simulink model "SWING_UP_ENERGY_BASED_plus_PP"  (R2022b)
settings: Solver=FixedStepAuto  StartTime=0.0  StopTime=inf  FixedStep=0.002  RelTol=1e-3  EnableMultiTasking=on
undefined symbols (not defined in the file or in its folder): A, B, C, D, g0, HIL, Ip, K, K_pp, L_kf, Lp, Lr, mp, mr, qc_get_step_size, Ra
libraries: quarc_library x8, simulink_extras x7
settings Model: ExtModeTrigDuration=10000  Creator=Utente  LastModifiedBy=Utente
settings SolverCC: AlgebraicLoopSolver=TrustRegion  PositivePriorityOrder=on
settings DataIOCC: ReturnWorkspaceOutputs=off
settings DebuggingCC: UnconnectedInputMsg=warning  UnconnectedOutputMsg=warning  UnconnectedLineMsg=warning  SFMachineParentedDataDiag=warning  ArithmeticOperatorsInVariantConditions=warning
settings ModelReferenceCC: EnableRefExpFcnMdlSchedulingChecks=on
settings SFSimCC: SimUseLocalCustomCode=off  CustomCodeUndefinedFunction=UseInterfaceOnly
settings RTWCC: Description=QUARC Win64 Target Using Toolchain  SystemTargetFile=quarc_win64.tlc  TemplateMakefile=quarc_default_tmf  RTWUseLocalCustomCode=off  Toolchain=QUARC win64 | nmake (64-bit Windows)  BuildConfiguration=Faster Runs
settings CodeAppCC: StateflowObjectComments=on
settings STFCustomTargetCC: TargetLangStandard=C99 (ISO)  ConcurrentExecutionCompliant=on  GRTInterface=on  UseToolchainInfoCompliant=on  SystemTargetFile=quarc_win64.tlc
settings GRTTargetCC: ParMdlRefBuildCompliant=off  CompOptLevelCompliant=off  CombineOutputUpdateFcns=off  MatFileLogging=off  CPPClassGenCompliant=off  GRTInterface=on  ExtMode=on  ExtModeMexFile=quarc_comm
settings ConfigComp: CovMetricSettings=dswe

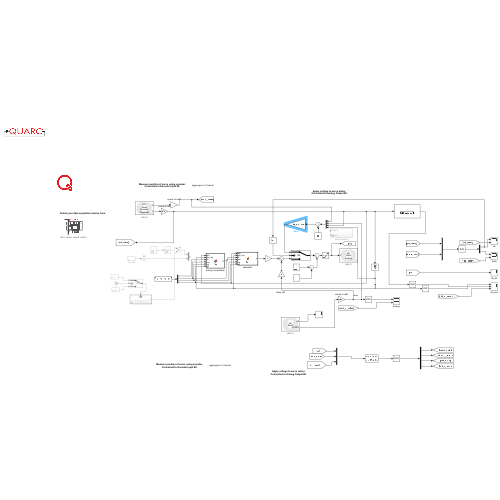
[thumbnail: Simulink's stored preview of the top-level diagram]
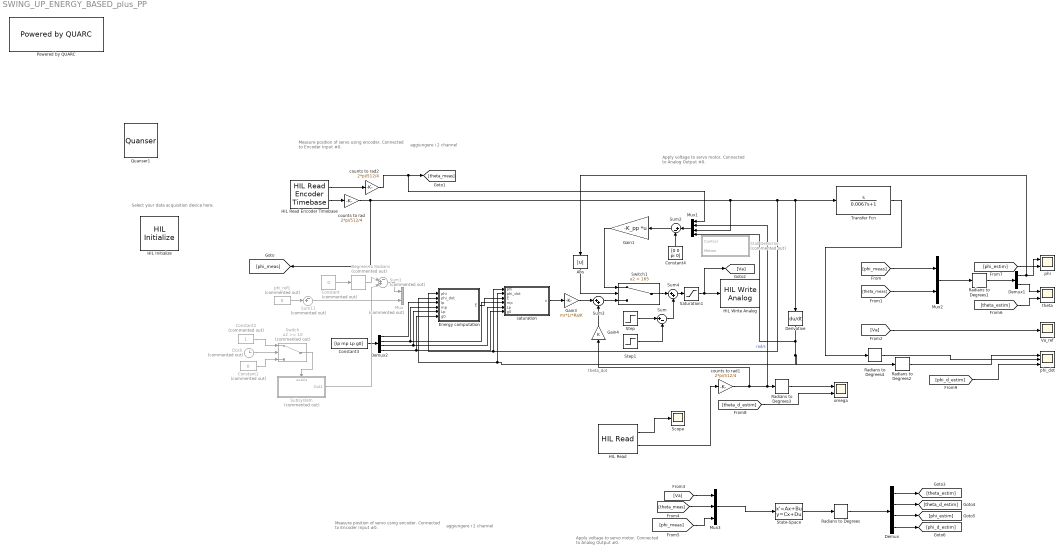
== system SWING_UP_ENERGY_BASED_plus_PP ==
  note: theta_dot
  note: aggiungere i 2 channel
  note: Apply voltage to servo motor.
      | Connected to Analog Output #0.
  note: Measure position of servo using encoder.
      | Connected to Encoder Input #0.
  note: aggiungere i 2 channel
  note: Measure position of servo using encoder.
      | Connected to Encoder Input #0.
  note: Apply voltage to servo motor.
      | Connected to Analog Output #0.
  note: Select your data acquisition device here.
  Abs : Abs  SaturateOnIntegerOverflow=off
  Clock : Clock  Commented=on
  Constant : Constant  Commented=on  Value=0
  Constant1 : Constant  Commented=on  Value=0
  Constant2 : Constant  Commented=on
  Constant3 : Constant  Value=[Ip mp Lp g0]
  Constant4 : Constant  Value=[0 0 pi 0]
  Degrees to Radians : simulink_extras/Transformations/Degrees to Radians  Commented=on
  Demux : Demux
  Demux1 : Demux  Outputs=2
  Demux2 : Demux
  Derivative : Derivative
  Energy computation : MATLAB Function  TreatAsAtomicUnit=on
  Gain1 : Gain  Gain=-K_pp  Multiplication=Matrix(K*u) (u vector)
  Gain3 : Gain  Gain=mr*Lr*Ra/K
  Gain4 : Gain  Gain=K
  HIL Initialize : quarc_library/Data Acquisition/Generic/Configuration/HIL Initialize  Priority=-99  object_name=HIL-1  board_type=qube_servo2_usb  board_number=0  board_options=""  exclusive=off  active=off  hardware_clocks=[0]  clock_modes=[]  initial_clock_frequencies=[]  set_clock_params_at_start=off  set_clock_params_at_switch_in=off  set_clock_frequencies_at_start=off  set_clock_frequencies_at_switch_in=off  analog_input_channels=[0]  analog_input_configurations=[]  analog_input_maximums=3  analog_input_minimums=-3  set_analog_input_params_at_start=off  set_analog_input_params_at_switch_in=off  analog_output_channels=[0]  analog_output_maximums=15  analog_output_minimums=-15  initial_analog_outputs=[0]  final_analog_outputs=[0]  watchdog_analog_outputs=0  set_analog_output_params_at_start=off  set_analog_output_params_at_switch_in=off  set_analog_outputs_at_start=on  set_analog_outputs_at_switch_in=off  set_analog_outputs_at_terminate=on  set_analog_outputs_at_switch_out=off  set_analog_outputs_on_watchdog=on  digital_input_channels=[]  digital_output_channels=[0]  digital_output_configuration=[]  initial_digital_outputs=[1]  final_digital_outputs=[0]  watchdog_digital_outputs=[0]  set_digital_output_params_at_start=off  set_digital_output_params_at_switch_in=off  set_digital_outputs_at_start=on  set_digital_outputs_at_switch_in=off  set_digital_outputs_at_terminate=on  set_digital_outputs_at_switch_out=off  set_digital_outputs_on_watchdog=on  encoder_channels=[0:1]  quadrature=[4]  encoder_filter_frequency=[]  initial_encoder_counts=[0]  set_encoder_params_at_start=off  set_encoder_params_at_switch_in=off  set_encoder_counts_at_start=on  set_encoder_counts_at_switch_in=off  pwm_channels=[]  pwm_modes=[]  pwm_frequency=[]  pwm_configuration=[]  pwm_alignment=[]  pwm_polarity=[]  pwm_leading_deadband=[]  pwm_trailing_deadband=[]  initial_pwm_outputs=[]  final_pwm_outputs=[]  watchdog_pwm_outputs=[]  set_pwm_params_at_start=off  set_pwm_params_at_switch_in=off  set_pwm_outputs_at_start=off  set_pwm_outputs_at_switch_in=off  set_pwm_outputs_at_terminate=off  set_pwm_outputs_at_switch_out=off  set_pwm_outputs_on_watchdog=off  other_output_channels=[11000:11002]  initial_other_outputs=[0 1 0]  final_other_outputs=[1 0 0]  watchdog_other_outputs=[0 0 1]  set_other_outputs_at_start=on  set_other_outputs_at_switch_in=off  set_other_outputs_at_terminate=on  set_other_outputs_at_switch_out=off  set_other_outputs_on_watchdog=on
  HIL Read : quarc_library/Data Acquisition/Generic/Immediate I//O/HIL Read  object_name=HIL-1  analog_channels=[0]  encoder_channels=[]  digital_channels=[]  other_channels=[14000]  sample_time=qc_get_step_size  active=on  vector_output=off  data_type_mode=Inherit via back propagation  encoder_data_type=double  digital_data_type=boolean
  HIL Read Encoder Timebase : quarc_library/Data Acquisition/Generic/Timebases/HIL Read Encoder Timebase  object_name=HIL-1  clock=0  channels=[0:1]  active=on  vector_output=off  data_type_mode=Inherit via back propagation  data_type=double  overflow_mode=Error on overflow  samples_in_buffer=max(ceil(1/qc_get_step_size), 1)
  HIL Write Analog : quarc_library/Data Acquisition/Generic/Immediate I//O/HIL Write Analog  object_name=HIL-1  channels=[0]  sample_time=-1  active=off  vector_input=off
  Mux : Mux  Commented=on  Inputs=2
  Mux1 : Mux
  Mux2 : Mux  Inputs=2
  Mux3 : Mux  Inputs=3
  Powered by QUARC : quarc_library/Logos/Powered by QUARC
  Quanser1 : quarc_library/Logos/Quanser
  Radians to Degrees{,1..4} (5 alike) : simulink_extras/Transformations/Radians to Degrees
  Saturation1 : Saturate  UpperLimit=10  LowerLimit=-10
  Scope : Scope
  Stall Detection : Subsystem  Commented=on
  State-Space : StateSpace  A=A-L_kf*C  B=[B-L_kf*D L_kf]  C=eye(4)  D=zeros(4,3)  InitialCondition=0
  Step : Step  SampleTime=0
  Step1 : Step  Time=1.001  SampleTime=0
  Subsystem : Subsystem  Commented=on
  Sum : Sum  Inputs=|+-
  Sum1 : Sum  Commented=on  Inputs=-++|
  Sum11 : Sum  Commented=on  Inputs=-+|
  Sum2 : Sum  Inputs=|+-
  Sum3 : Sum  Inputs=|++
  Sum4 : Sum  Inputs=|++
  Switch : Switch  Commented=on  Threshold=10  SaturateOnIntegerOverflow=off  InputSameDT=off
  Switch1 : Switch  Criteria=u2 > Threshold  Threshold=165  SaturateOnIntegerOverflow=off  InputSameDT=off
  Transfer Fcn : TransferFcn  Numerator=[1 0]  Denominator=[0.0067 1]
  Va_ref : Scope
  counts to rad : Gain  Gain=2*pi/512/4
  counts to rad1 : Gain  Gain=2*pi/512/4
  counts to rad2 : Gain  Gain=2*pi/512/4
  omega : Scope  NumInputPorts=2
  phi : Scope  NumInputPorts=2
  phi_dot : Scope  NumInputPorts=3
  phi_ref1 : Constant  Commented=on  Value=0
  saturation : MATLAB Function  TreatAsAtomicUnit=on
  theta : Scope  NumInputPorts=2
  wires:
  [Va] -> Mux3/1
  Demux2/3 -> saturation/5(Lp), Energy computation/5(Lp)
  Demux2/2 -> saturation/4(mp), Energy computation/4(mp)
  saturation/1(u) -> Gain3/1
  Radians to Degrees3/1 -> omega/1
  Demux2/4 -> Energy computation/6(g0), saturation/6(g0)
  Demux2/1 -> Energy computation/3(Ip)
  counts to rad2/1 -> Mux1/1, [theta_meas]
  Radians to Degrees1/1 -> Demux1/1
  Constant3/1 -> Demux2/1
  counts to rad/1 -> [phi_meas], Mux1/3, Energy computation/1(phi), saturation/1(phi), Derivative/1, Transfer Fcn/1
  Energy computation/1(E) -> saturation/3(E)
  Clock/1 -> Switch/2
  Demux/1 -> [theta_estim]
  Gain4/1 -> Sum3/2
  Saturation1/1 -> [Va], HIL Write Analog/1
  Constant1/1 -> Switch/3
  Switch/1 -> Subsystem/Enable
  Sum1/1 -> Mux/1
  Radians to Degrees4/1 -> phi_dot/2
  Demux/3 -> [phi_estim]
  [phi_d_estim] -> phi_dot/3
  [phi_meas] -> Mux3/3
  [theta_d_estim] -> omega/2
  [theta_estim] -> theta/2
  HIL Read/2 -> counts to rad1/1
  Radians to Degrees2/1 -> phi_dot/1
  [theta_meas] -> Mux3/2
  Demux1/2 -> theta/1
  HIL Read/1 -> Scope/1
  Constant/1 -> Degrees to Radians/1
  [theta_meas] -> Mux2/2
  Transfer Fcn/1 -> Radians to Degrees4/1
  Degrees to Radians/1 -> Sum1/2
  Demux1/1 -> Abs/1, phi/1
  State-Space/1 -> Radians to Degrees/1
  Sum11/1 -> Mux/2
  [phi_meas] -> Mux2/1
  Mux2/1 -> Radians to Degrees1/1
  phi_ref1/1 -> Sum11/2
  Subsystem/1(Out1) -> Sum1/3
  Constant2/1 -> Switch/1
  Mux3/1 -> State-Space/1
  HIL Read Encoder Timebase/1 -> counts to rad2/1
  Demux/4 -> [phi_d_estim]
  [phi_estim] -> phi/2
  [Va] -> Va_ref/1
  Radians to Degrees/1 -> Demux/1
  Derivative/1 -> Mux1/4, Energy computation/2(phi_dot), saturation/2(phi_dot), Radians to Degrees2/1
  counts to rad1/1 -> Gain4/1, Mux1/2, Radians to Degrees3/1  "rad/s"
  Demux/2 -> [theta_d_estim]
  Gain3/1 -> Sum3/1
  HIL Read Encoder Timebase/2 -> counts to rad/1
  Abs/1 -> Switch1/2
  Sum3/1 -> Switch1/3
  Sum2/1 -> Gain1/1
  Constant4/1 -> Sum2/2
  Gain1/1 -> Switch1/1
  Mux1/1 -> Sum2/1
  Step/1 -> Sum/1
  Step1/1 -> Sum/2
  Sum4/1 -> Saturation1/1
  Switch1/1 -> Sum4/1
  Sum/1 -> Sum4/2

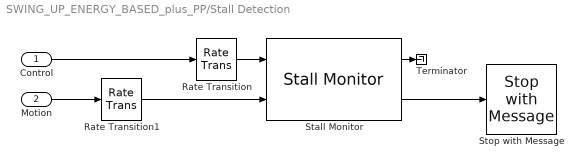
== system SWING_UP_ENERGY_BASED_plus_PP/Stall Detection ==
  Control : Inport
  Motion : Inport  Port=2
  Rate Transition : RateTransition
  Rate Transition1 : RateTransition
  Stall Monitor : quarc_library/Discrete/Stall Monitor  control_threshold=5  motion_threshold=0.3  duration_s=20
      settings: SourceProductName=QUARC Targets
  Stop with Message : quarc_library/Sinks/Error Handling/Stop with Message  message_type=Fixed error message  message_icon=Error  message=Stall Detected! Please ensure that the DC motor is free to move and is functioning properly
  Terminator : Terminator
  wires:
  Control/1 -> Rate Transition/1
  Motion/1 -> Rate Transition1/1
  Stall Monitor/2 -> Stop with Message/1
  Stall Monitor/1 -> Terminator/1
  Rate Transition/1 -> Stall Monitor/1
  Rate Transition1/1 -> Stall Monitor/2

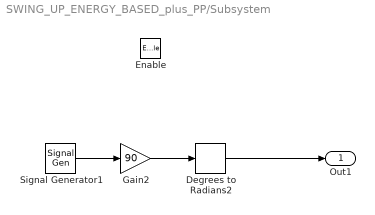
== system SWING_UP_ENERGY_BASED_plus_PP/Subsystem ==
  Enable : EnablePort
  Degrees to Radians2 : simulink_extras/Transformations/Degrees to Radians
  Gain2 : Gain  Gain=90
  Signal Generator1 : SignalGenerator  Frequency=0.05
  Out1 : Outport
  wires:
  Signal Generator1/1 -> Gain2/1
  Degrees to Radians2/1 -> Out1/1
  Gain2/1 -> Degrees to Radians2/1

== matlab function SWING_UP_ENERGY_BASED_plus_PP/Energy computation ==
  data: phi input; E output; phi_dot input; Ip input; mp input; Lp input; g0 input
function E = fcn(phi, phi_dot, Ip, mp, Lp, g0)
E = 0.5*Ip*phi_dot^2 + 0.5*mp*Lp*g0*(1-cos(phi));

== matlab function SWING_UP_ENERGY_BASED_plus_PP/saturation ==
  data: phi input; u output; phi_dot input; E input; mp input; Lp input; g0 input
function u = fcn(phi, phi_dot, E, mp, Lp, g0)
mu = 30;
Er = 0.5*mp*Lp*g0*(1-cos(pi));  
u = mu*(Er- E)*sign(phi_dot*cos(phi));
